simulink model "HANcoder_E407_GTSync_v3"  (R2018b)
settings: Solver=FixedStepDiscrete  StartTime=0.0  StopTime=1  FixedStep=0.01  RelTol=1e-3
PreLoadFcn:
  | librarySetup
  | eval([bdroot,'_startup']) %Calling [modelName]_startup.m
values from neighbouring files (symbols this model uses):
  frequency_IRQ = 100    [HANcoder_E407_GTSync_startup.m]    (also in HANcoder_E407_GTSync_v3_clean_startup.m = 99; HANcoder_E407_GTSync_v3_startup.m = 99)
  HANtuneOverride = Simulink.Parameter    [HANcoder_E407_GTSync_startup.m]    (also in HANcoder_E407_GTSync_v3_clean_startup.m; HANcoder_E407_GTSync_v3_startup.m)
  LED_ticks_toggle = 10000    [HANcoder_E407_GTSync_startup.m]    (also in HANcoder_E407_GTSync_v3_clean_startup.m; HANcoder_E407_GTSync_v3_startup.m)
  Master_Role = 1    [HANcoder_E407_GTSync_v3_clean_startup.m]    (also in HANcoder_E407_GTSync_v3_startup.m)
  matrix_rows = 2    [HANcoder_E407_GTSync_v3_clean_startup.m]    (also in HANcoder_E407_GTSync_v3_startup.m)
  Sync_ID = 1    [HANcoder_E407_GTSync_v3_clean_startup.m]    (also in HANcoder_E407_GTSync_v3_startup.m)
  time_difference_threshold = 500    [HANcoder_E407_GTSync_v3_clean_startup.m]    (also in HANcoder_E407_GTSync_v3_startup.m = 100)
  TM0 = 100    [HANcoder_E407_GTSync_v3_clean_startup.m]    (also in HANcoder_E407_GTSync_v3_startup.m = 0)
  TM1 = 20000    [HANcoder_E407_GTSync_v3_clean_startup.m]    (also in HANcoder_E407_GTSync_v3_startup.m = 25000)
  TM2 = 30000    [HANcoder_E407_GTSync_v3_clean_startup.m]    (also in HANcoder_E407_GTSync_v3_startup.m = 37500)
  TM3 = 40000    [HANcoder_E407_GTSync_v3_clean_startup.m]    (also in HANcoder_E407_GTSync_v3_startup.m)
  Vote1_ID = 12    [HANcoder_E407_GTSync_v3_clean_startup.m]    (also in HANcoder_E407_GTSync_v3_startup.m)
  Vote2_ID = 22    [HANcoder_E407_GTSync_v3_clean_startup.m]    (also in HANcoder_E407_GTSync_v3_startup.m)
  Vote3_ID = 32    [HANcoder_E407_GTSync_v3_clean_startup.m]    (also in HANcoder_E407_GTSync_v3_startup.m)
undefined symbols (not defined in the file or in its folder): votes
libraries: HANcoder_STM32_Target x20, simulink x3, simulink_extras x1
(part 2 of 2)

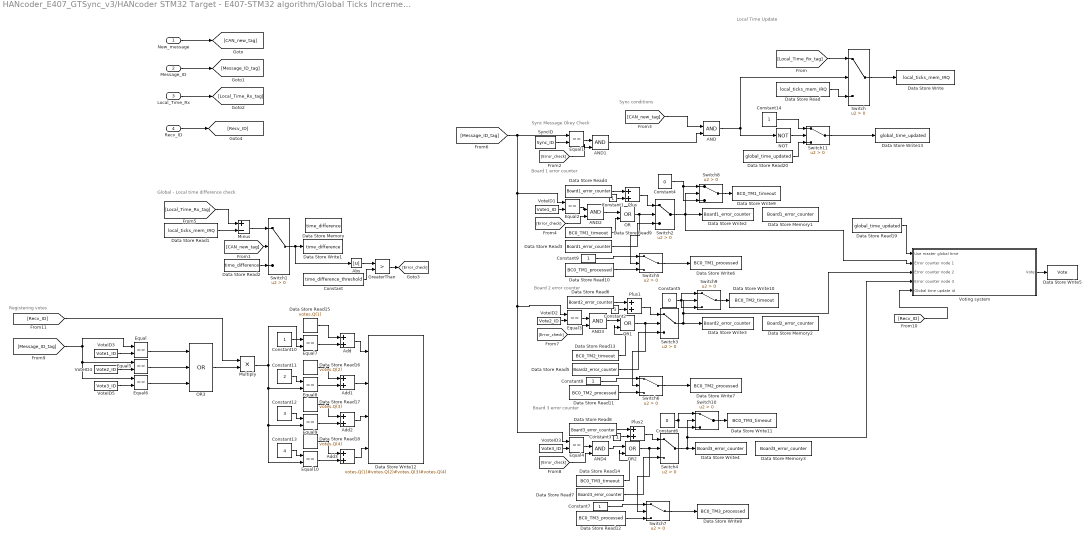
== system HANcoder_E407_GTSync_v3/HANcoder STM32 Target - E407-STM32 algorithm/Global Ticks Increment/CAN Management/Received message processing ==
  note: Registering votes
  note: Board 3 error counter
  note: Board 2 error counter
  note: Board 1 error counter
  note: Sync Message Okey Check
  note: Sync conditions
  note: Global - Local time difference check
  note: Local Time Update
  New_message : Inport
  Message_ID : Inport  Port=2
  Local_Time_Rx : Inport  Port=3
  Recv_ID : Inport  Port=4
  AND{,1..4} (5 alike) : Logic  IconShape=distinctive  AllPortsSameDT=off  OutDataTypeStr=boolean
  Abs : Abs
  Add{,1..3} (4 alike) : Sum
  Constant : Constant  Value=time_difference_threshold
  Constant{1..3,7..10,14} (8 alike) : Constant
  Constant11 : Constant  Value=2
  Constant12 : Constant  Value=3
  Constant13 : Constant  Value=4
  Constant4 : Constant  Value=0
  Constant5 : Constant  Value=0
  Constant6 : Constant  Value=0
  Data Store Memory : DataStoreMemory  DataStoreName=time_difference  ReadBeforeWriteMsg=warning  WriteAfterWriteMsg=warning  WriteAfterReadMsg=warning  ShowAdditionalParam=off
  Data Store Memory1 : DataStoreMemory  DataStoreName=Board1_error_counter  ReadBeforeWriteMsg=warning  WriteAfterWriteMsg=warning  WriteAfterReadMsg=warning  ShowAdditionalParam=off  OutMin=0  OutMax=4294967294  OutDataTypeStr=uint32
  Data Store Memory2 : DataStoreMemory  DataStoreName=Board2_error_counter  ReadBeforeWriteMsg=warning  WriteAfterWriteMsg=warning  WriteAfterReadMsg=warning  ShowAdditionalParam=off  OutMin=0  OutMax=4294967294  OutDataTypeStr=uint32
  Data Store Memory3 : DataStoreMemory  DataStoreName=Board3_error_counter  ReadBeforeWriteMsg=warning  WriteAfterWriteMsg=warning  WriteAfterReadMsg=warning  ShowAdditionalParam=off  OutMin=0  OutMax=4294967294  OutDataTypeStr=uint32
  Data Store Read : DataStoreRead  DataStoreName=local_ticks_mem_IRQ
  Data Store Read1 : DataStoreRead  DataStoreName=local_ticks_mem_IRQ
  Data Store Read10 : DataStoreRead  DataStoreName=BC0_TM1_processed
  Data Store Read11 : DataStoreRead  DataStoreName=BC0_TM2_processed
  Data Store Read12 : DataStoreRead  DataStoreName=BC0_TM3_processed
  Data Store Read13 : DataStoreRead  DataStoreName=BC0_TM2_timeout
  Data Store Read14 : DataStoreRead  DataStoreName=BC0_TM3_timeout
  Data Store Read15 : DataStoreRead  DataStoreName=votes  DataStoreElements=votes.Q(1)
  Data Store Read16 : DataStoreRead  DataStoreName=votes  DataStoreElements=votes.Q(2)
  Data Store Read17 : DataStoreRead  DataStoreName=votes  DataStoreElements=votes.Q(3)
  Data Store Read18 : DataStoreRead  DataStoreName=votes  DataStoreElements=votes.Q(4)
  Data Store Read19 : DataStoreRead  DataStoreName=global_time_updated
  Data Store Read2 : DataStoreRead  DataStoreName=time_difference
  Data Store Read20 : DataStoreRead  DataStoreName=global_time_updated
  Data Store Read3 : DataStoreRead  DataStoreName=Board1_error_counter
  Data Store Read4 : DataStoreRead  DataStoreName=Board1_error_counter
  Data Store Read5 : DataStoreRead  DataStoreName=Board2_error_counter
  Data Store Read6 : DataStoreRead  DataStoreName=Board2_error_counter
  Data Store Read7 : DataStoreRead  DataStoreName=Board3_error_counter
  Data Store Read8 : DataStoreRead  DataStoreName=Board3_error_counter
  Data Store Read9 : DataStoreRead  DataStoreName=BC0_TM1_timeout
  Data Store Write : DataStoreWrite  DataStoreName=local_ticks_mem_IRQ
  Data Store Write1 : DataStoreWrite  DataStoreName=time_difference
  Data Store Write10 : DataStoreWrite  DataStoreName=BC0_TM2_timeout
  Data Store Write11 : DataStoreWrite  DataStoreName=BC0_TM3_timeout
  Data Store Write12 : DataStoreWrite  DataStoreName=votes  DataStoreElements=votes.Q(1)#votes.Q(2)#votes.Q(3)#votes.Q(4)
  Data Store Write13 : DataStoreWrite  DataStoreName=global_time_updated
  Data Store Write2 : DataStoreWrite  DataStoreName=Board1_error_counter
  Data Store Write3 : DataStoreWrite  DataStoreName=Board2_error_counter
  Data Store Write4 : DataStoreWrite  DataStoreName=Board3_error_counter
  Data Store Write5 : DataStoreWrite  DataStoreName=Vote
  Data Store Write6 : DataStoreWrite  DataStoreName=BC0_TM1_processed
  Data Store Write7 : DataStoreWrite  DataStoreName=BC0_TM2_processed
  Data Store Write8 : DataStoreWrite  DataStoreName=BC0_TM3_processed
  Data Store Write9 : DataStoreWrite  DataStoreName=BC0_TM1_timeout
  Equal{,1..10} (11 alike) : RelationalOperator  Operator===  OutDataTypeStr=boolean  RndMeth=Simplest
  GreaterThan : RelationalOperator  Operator=>  OutDataTypeStr=boolean  RndMeth=Simplest
  Minus : Sum  Inputs=+-
  Multiply : Product
  NOT : Logic  Operator=NOT  IconShape=distinctive  AllPortsSameDT=off  OutDataTypeStr=boolean
  OR : Logic  Operator=OR  IconShape=distinctive  AllPortsSameDT=off  OutDataTypeStr=boolean
  OR1 : Logic  Operator=OR  IconShape=distinctive  AllPortsSameDT=off  OutDataTypeStr=boolean
  OR2 : Logic  Operator=OR  IconShape=distinctive  AllPortsSameDT=off  OutDataTypeStr=boolean
  OR3 : Logic  Operator=OR  Inputs=3  IconShape=distinctive  AllPortsSameDT=off  OutDataTypeStr=boolean
  Plus : Sum
  Plus1 : Sum
  Plus2 : Sum
  Switch{,1..11} (12 alike) : Switch  Criteria=u2 > Threshold
  SyncID : Constant  Value=Sync_ID
  VosteID3 : Constant  Value=Vote3_ID
  VoteID1 : Constant  Value=Vote1_ID
  VoteID2 : Constant  Value=Vote2_ID
  VoteID3 : Constant  Value=Vote1_ID
  VoteID4 : Constant  Value=Vote2_ID
  VoteID5 : Constant  Value=Vote3_ID
  Voting system : Subsystem
  wires:
  Data Store Read/1 -> Switch/3
  AND/1 -> Switch/2, NOT/1
  Switch/1 -> Data Store Write/1
  New_message/1 -> [CAN_new_tag]
  Message_ID/1 -> [Message_ID_tag]
  Local_Time_Rx/1 -> [Local_Time_Rx_tag]
  [Local_Time_Rx_tag] -> Switch/1
  AND1/1 -> AND/2
  [CAN_new_tag] -> AND/1
  [Local_Time_Rx_tag] -> Minus/1
  Data Store Read1/1 -> Minus/2
  Minus/1 -> Switch1/1
  [CAN_new_tag] -> Switch1/2
  Data Store Read2/1 -> Switch1/3
  SyncID/1 -> Equal1/2
  VoteID1/1 -> Equal2/2
  VoteID2/1 -> Equal3/2
  VosteID3/1 -> Equal4/2
  [Message_ID_tag] -> Equal4/1, Equal3/1, Equal2/1, Equal1/1
  Equal1/1 -> AND1/1
  Switch1/1 -> Abs/1, Data Store Write1/1
  Abs/1 -> GreaterThan/1
  Constant/1 -> GreaterThan/2
  [Error_check] -> AND1/2
  GreaterThan/1 -> [Error_check]
  Equal2/1 -> AND2/1
  [Error_check] -> AND2/2
  [Error_check] -> AND3/2
  Equal3/1 -> AND3/1
  [Error_check] -> AND4/2
  Equal4/1 -> AND4/1
  Data Store Read3/1 -> Switch2/3
  Data Store Read4/1 -> Plus/1
  Constant1/1 -> Plus/2
  Plus/1 -> Switch2/1
  Plus1/1 -> Switch3/1
  Constant2/1 -> Plus1/2
  Data Store Read6/1 -> Plus1/1
  Data Store Read5/1 -> Switch3/3
  Data Store Read7/1 -> Switch4/3
  Data Store Read8/1 -> Plus2/1
  Constant3/1 -> Plus2/2
  Plus2/1 -> Switch4/1
  Switch2/1 -> Voting system/2(Error counter node 1), Switch8/2, Data Store Write2/1
  Voting system/1(Vote) -> Data Store Write5/1
  [Recv_ID] -> Voting system/5(Global time update id)
  Recv_ID/1 -> [Recv_ID]
  Switch5/1 -> Data Store Write6/1
  AND3/1 -> OR1/1
  Switch6/1 -> Data Store Write7/1
  Data Store Read12/1 -> Switch7/3
  Switch7/1 -> Data Store Write8/1
  OR/1 -> Switch5/2, Switch2/2
  AND2/1 -> OR/1
  Data Store Read9/1 -> OR/2
  Constant4/1 -> Switch8/3, Switch8/1
  Switch8/1 -> Data Store Write9/1
  OR1/1 -> Switch6/2, Switch3/2
  Data Store Read13/1 -> OR1/2
  Switch3/1 -> Switch9/2, Voting system/3(Error counter node 2), Data Store Write3/1
  Switch9/1 -> Data Store Write10/1
  Constant5/1 -> Switch9/1, Switch9/3
  Switch10/1 -> Data Store Write11/1
  Switch4/1 -> Voting system/4(Error counter node 3), Switch10/2, Data Store Write4/1
  Constant6/1 -> Switch10/1, Switch10/3
  Data Store Read14/1 -> OR2/2
  OR2/1 -> Switch7/2, Switch4/2
  AND4/1 -> OR2/1
  Constant7/1 -> Switch7/1
  Data Store Read11/1 -> Switch6/3
  Constant8/1 -> Switch6/1
  Data Store Read10/1 -> Switch5/3
  Constant9/1 -> Switch5/1
  Equal/1 -> OR3/1
  VoteID3/1 -> Equal/2
  [Message_ID_tag] -> Equal/1, Equal6/1, Equal5/1
  VoteID4/1 -> Equal5/2
  Equal5/1 -> OR3/2
  VoteID5/1 -> Equal6/2
  Equal6/1 -> OR3/3
  [Recv_ID] -> Multiply/1
  OR3/1 -> Multiply/2
  Constant10/1 -> Equal7/1
  Equal7/1 -> Add/2
  Add/1 -> Data Store Write12/1
  Data Store Read15/1 -> Add/1
  Data Store Read16/1 -> Add1/1
  Constant11/1 -> Equal8/1
  Equal8/1 -> Add1/2
  Add1/1 -> Data Store Write12/2
  Equal9/1 -> Add2/2
  Data Store Read17/1 -> Add2/1
  Constant12/1 -> Equal9/1
  Add2/1 -> Data Store Write12/3
  Data Store Read18/1 -> Add3/1
  Multiply/1 -> Equal10/2, Equal9/2, Equal8/2, Equal7/2
  Equal10/1 -> Add3/2
  Constant13/1 -> Equal10/1
  Add3/1 -> Data Store Write12/4
  Data Store Read19/1 -> Voting system/1(Use master global time)
  NOT/1 -> Switch11/2
  Switch11/1 -> Data Store Write13/1
  Data Store Read20/1 -> Switch11/3
  Constant14/1 -> Switch11/1

== system HANcoder_E407_GTSync_v3/HANcoder STM32 Target - E407-STM32 algorithm/Global Ticks Increment/Send/CAN send ==
  In1 : Inport
  In2 : Inport  Port=2
  In3 : Inport  Port=3
  In4 : Inport  Port=4
  In5 : Inport  Port=5
  In6 : Inport  Port=6
  In7 : Inport  Port=7
  In8 : Inport  Port=8
  In9 : Inport  Port=9
  S-Function : M-S-Function  FunctionName=sfcn_can_send  Parameters=tsamp, canBus, frameType, inputNumber, dataType, byteOrder
  wires:
  In1/1 -> S-Function/1
  In2/1 -> S-Function/2
  In3/1 -> S-Function/3
  In4/1 -> S-Function/4
  In5/1 -> S-Function/5
  In6/1 -> S-Function/6
  In7/1 -> S-Function/7
  In8/1 -> S-Function/8
  In9/1 -> S-Function/9

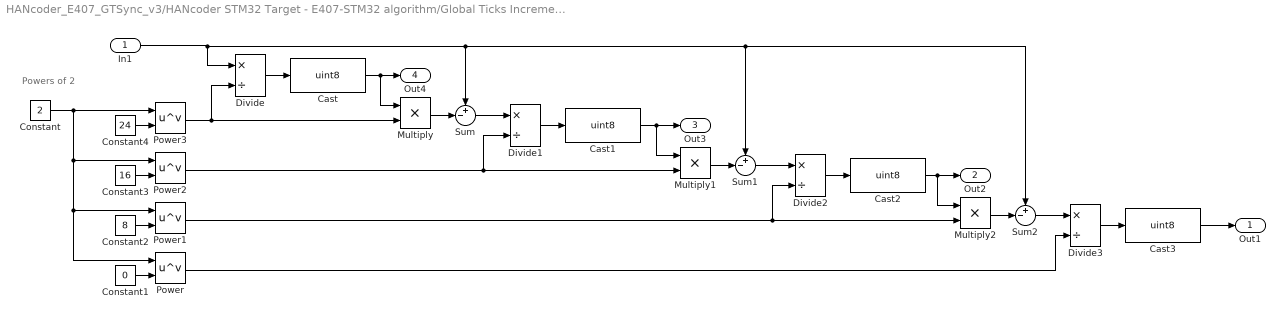
== system HANcoder_E407_GTSync_v3/HANcoder STM32 Target - E407-STM32 algorithm/Global Ticks Increment/Send/UINT32 to UINT8 ==
  note: Powers of 2
  In1 : Inport
  Cast{,1..3} (4 alike) : DataTypeConversion  OutDataTypeStr=uint8
  Constant : Constant  Value=2
  Constant1 : Constant  Value=0
  Constant2 : Constant  Value=8
  Constant3 : Constant  Value=16
  Constant4 : Constant  Value=24
  Divide{,1..3} (4 alike) : Product  Inputs=*/
  Multiply : Product
  Multiply1 : Product
  Multiply2 : Product
  Power{,1..3} (4 alike) : Math  Operator=pow  SaturateOnIntegerOverflow=on
  Sum : Sum  Inputs=+-|
  Sum1 : Sum  Inputs=+-|
  Sum2 : Sum  Inputs=+-|
  Out1 : Outport
  Out2 : Outport  Port=2
  Out3 : Outport  Port=3
  Out4 : Outport  Port=4
  wires:
  Constant2/1 -> Power1/2
  Constant3/1 -> Power2/2
  Constant4/1 -> Power3/2
  Power2/1 -> Multiply1/2, Divide1/2
  Constant1/1 -> Power/2
  Power3/1 -> Divide/2, Multiply/2
  Constant/1 -> Power/1, Power1/1, Power2/1, Power3/1
  Divide/1 -> Cast/1
  Cast/1 -> Multiply/1, Out4/1
  Multiply/1 -> Sum/2
  Divide1/1 -> Cast1/1
  Sum/1 -> Divide1/1
  Cast1/1 -> Out3/1, Multiply1/1
  Multiply1/1 -> Sum1/2
  Multiply2/1 -> Sum2/2
  Cast2/1 -> Out2/1, Multiply2/1
  Divide2/1 -> Cast2/1
  Power1/1 -> Multiply2/2, Divide2/2
  Sum1/1 -> Divide2/1
  Sum2/1 -> Divide3/1
  In1/1 -> Sum1/1, Sum2/1, Sum/1, Divide/1
  Power/1 -> Divide3/2
  Divide3/1 -> Cast3/1
  Cast3/1 -> Out1/1

== system HANcoder_E407_GTSync_v3/HANcoder STM32 Target - E407-STM32 algorithm/Global Ticks Increment/CAN Management/CAN Recieve/CAN receive ==
  In1 : Inport
  Enabled Subsystem : Subsystem  TreatAsAtomicUnit=on
  S-Function : M-S-Function  FunctionName=sfcn_can_receive  Parameters=tsamp, canBus, outputNumber, dataType, byteOrder
  Out1 : Outport
  Out2 : Outport  Port=2
  Out3 : Outport  Port=3
  Out4 : Outport  Port=4
  Out5 : Outport  Port=5
  Out6 : Outport  Port=6
  Out7 : Outport  Port=7
  Out8 : Outport  Port=8
  Out9 : Outport  Port=9
  wires:
  S-Function/9 -> Enabled Subsystem/8(In8)
  S-Function/4 -> Enabled Subsystem/3(In3)
  S-Function/5 -> Enabled Subsystem/4(In4)
  S-Function/8 -> Enabled Subsystem/7(In7)
  S-Function/7 -> Enabled Subsystem/6(In6)
  S-Function/6 -> Enabled Subsystem/5(In5)
  Enabled Subsystem/8(Out8) -> Out9/1
  Enabled Subsystem/7(Out7) -> Out8/1
  Enabled Subsystem/6(Out6) -> Out7/1
  Enabled Subsystem/5(Out5) -> Out6/1
  Enabled Subsystem/4(Out4) -> Out5/1
  Enabled Subsystem/3(Out3) -> Out4/1
  Enabled Subsystem/2(Out2) -> Out3/1
  Enabled Subsystem/1(Out1) -> Out2/1
  S-Function/3 -> Enabled Subsystem/2(In2)
  S-Function/2 -> Enabled Subsystem/1(In1)
  S-Function/1 -> Out1/1, Enabled Subsystem/Enable
  In1/1 -> S-Function/1

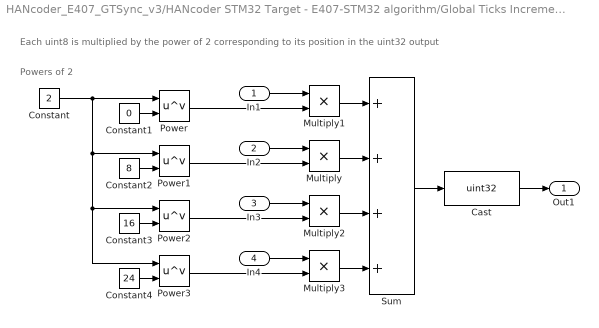
== system HANcoder_E407_GTSync_v3/HANcoder STM32 Target - E407-STM32 algorithm/Global Ticks Increment/CAN Management/CAN Recieve/UINT8 to UINT32 ==
  note: Each uint8 is multiplied by the power of 2 corresponding to its position in the uint32 output
  note: Powers of 2
  In1 : Inport
  In2 : Inport  Port=2
  In3 : Inport  Port=3
  In4 : Inport  Port=4
  Cast : DataTypeConversion  OutDataTypeStr=uint32
  Constant : Constant  Value=2
  Constant1 : Constant  Value=0
  Constant2 : Constant  Value=8
  Constant3 : Constant  Value=16
  Constant4 : Constant  Value=24
  Multiply{,1..3} (4 alike) : Product
  Power{,1..3} (4 alike) : Math  Operator=pow  SaturateOnIntegerOverflow=on
  Sum : Sum  Inputs=++++
  Out1 : Outport
  wires:
  Cast/1 -> Out1/1
  Sum/1 -> Cast/1
  In1/1 -> Multiply1/1
  In2/1 -> Multiply/1
  In3/1 -> Multiply2/1
  In4/1 -> Multiply3/1
  Constant/1 -> Power3/1, Power2/1, Power1/1, Power/1
  Constant1/1 -> Power/2
  Constant2/1 -> Power1/2
  Constant3/1 -> Power2/2
  Constant4/1 -> Power3/2
  Power/1 -> Multiply1/2
  Power1/1 -> Multiply/2
  Power2/1 -> Multiply2/2
  Power3/1 -> Multiply3/2
  Multiply3/1 -> Sum/4
  Multiply2/1 -> Sum/3
  Multiply/1 -> Sum/2
  Multiply1/1 -> Sum/1

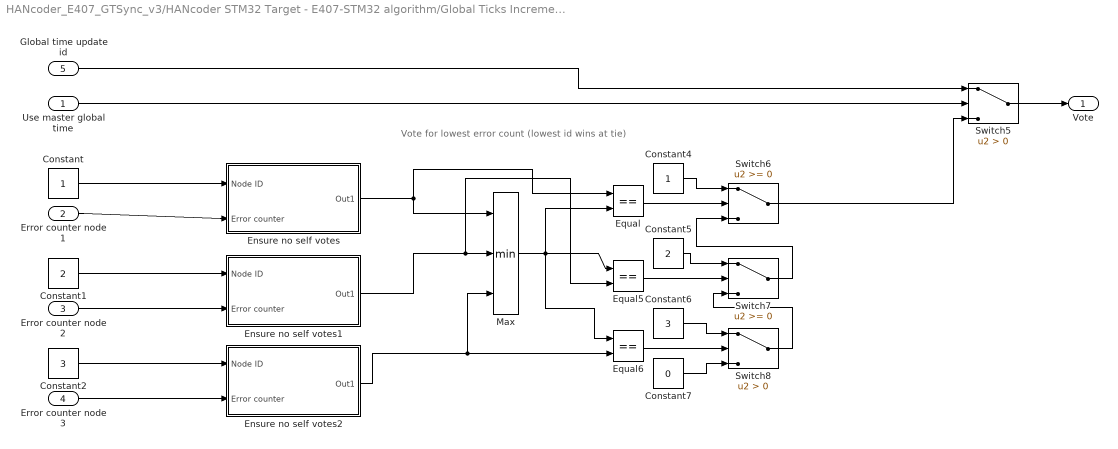
== system HANcoder_E407_GTSync_v3/HANcoder STM32 Target - E407-STM32 algorithm/Global Ticks Increment/CAN Management/Received message processing/Voting system ==
  note: Vote for lowest error count (lowest id wins at tie)
  Use master global time : Inport
  Error counter node 1 : Inport  Port=2
  Error counter node 2 : Inport  Port=3
  Error counter node 3 : Inport  Port=4
  Global time update id : Inport  Port=5
  Constant : Constant
  Constant1 : Constant  Value=2
  Constant2 : Constant  Value=3
  Constant4 : Constant
  Constant5 : Constant  Value=2
  Constant6 : Constant  Value=3
  Constant7 : Constant  Value=0
  Ensure no self votes : Subsystem
  Ensure no self votes1 : Subsystem
  Ensure no self votes2 : Subsystem
  Equal : RelationalOperator  Operator===  OutDataTypeStr=boolean  RndMeth=Simplest
  Equal5 : RelationalOperator  Operator===  OutDataTypeStr=boolean  RndMeth=Simplest
  Equal6 : RelationalOperator  Operator===  OutDataTypeStr=boolean  RndMeth=Simplest
  Max : MinMax  Inputs=3
  Switch5 : Switch  Criteria=u2 > Threshold
  Switch6 : Switch
  Switch7 : Switch
  Switch8 : Switch  Criteria=u2 > Threshold
  Vote : Outport
  wires:
  Equal5/1 -> Switch7/2
  Ensure no self votes1/1(Out1) -> Equal5/2, Max/2
  Constant5/1 -> Switch7/1
  Equal6/1 -> Switch8/2
  Ensure no self votes2/1(Out1) -> Max/3, Equal6/2
  Switch7/1 -> Switch6/3
  Switch5/1 -> Vote/1
  Max/1 -> Equal/2, Equal5/1, Equal6/1
  Switch6/1 -> Switch5/3
  Switch8/1 -> Switch7/3
  Constant7/1 -> Switch8/3
  Equal/1 -> Switch6/2
  Constant6/1 -> Switch8/1
  Constant4/1 -> Switch6/1
  Global time update id/1 -> Switch5/1
  Use master global time/1 -> Switch5/2
  Ensure no self votes/1(Out1) -> Equal/1, Max/1
  Constant/1 -> Ensure no self votes/1(Node ID)
  Error counter node 1/1 -> Ensure no self votes/2(Error counter)
  Error counter node 2/1 -> Ensure no self votes1/2(Error counter)
  Constant1/1 -> Ensure no self votes1/1(Node ID)
  Error counter node 3/1 -> Ensure no self votes2/2(Error counter)
  Constant2/1 -> Ensure no self votes2/1(Node ID)

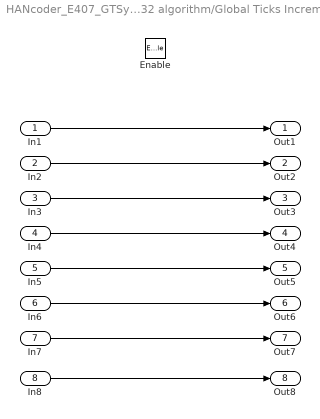
== system HANcoder_E407_GTSync_v3/HANcoder STM32 Target - E407-STM32 algorithm/Global Ticks Increment/CAN Management/CAN Recieve/CAN receive/Enabled Subsystem ==
  In1 : Inport
  In2 : Inport  Port=2
  In3 : Inport  Port=3
  In4 : Inport  Port=4
  In5 : Inport  Port=5
  In6 : Inport  Port=6
  In7 : Inport  Port=7
  In8 : Inport  Port=8
  Enable : EnablePort
  Out1 : Outport
  Out2 : Outport  Port=2
  Out3 : Outport  Port=3
  Out4 : Outport  Port=4
  Out5 : Outport  Port=5
  Out6 : Outport  Port=6
  Out7 : Outport  Port=7
  Out8 : Outport  Port=8
  wires:
  In8/1 -> Out8/1
  In7/1 -> Out7/1
  In6/1 -> Out6/1
  In5/1 -> Out5/1
  In4/1 -> Out4/1
  In3/1 -> Out3/1
  In2/1 -> Out2/1
  In1/1 -> Out1/1

== system HANcoder_E407_GTSync_v3/HANcoder STM32 Target - E407-STM32 algorithm/Global Ticks Increment/CAN Management/Received message processing/Voting system/Ensure no self votes ==
  Node ID : Inport
  Error counter : Inport  Port=2
  Data Store Read : DataStoreRead  DataStoreName=Board_ID
  Equal1 : RelationalOperator  Operator===  OutDataTypeStr=boolean  RndMeth=Simplest
  MAX error count : Constant  Value=4294967295  OutDataTypeStr=uint32
  Switch : Switch  Criteria=u2 > Threshold
  Out1 : Outport
  wires:
  Equal1/1 -> Switch/2
  Data Store Read/1 -> Equal1/2
  MAX error count/1 -> Switch/1
  Switch/1 -> Out1/1
  Error counter/1 -> Switch/3
  Node ID/1 -> Equal1/1

== system HANcoder_E407_GTSync_v3/HANcoder STM32 Target - E407-STM32 algorithm/Global Ticks Increment/CAN Management/Received message processing/Voting system/Ensure no self votes1 ==
  Node ID : Inport
  Error counter : Inport  Port=2
  Data Store Read : DataStoreRead  DataStoreName=Board_ID
  Equal1 : RelationalOperator  Operator===  OutDataTypeStr=boolean  RndMeth=Simplest
  MAX error count : Constant  Value=4294967295  OutDataTypeStr=uint32
  Switch : Switch  Criteria=u2 > Threshold
  Out1 : Outport
  wires:
  Equal1/1 -> Switch/2
  Data Store Read/1 -> Equal1/2
  MAX error count/1 -> Switch/1
  Switch/1 -> Out1/1
  Error counter/1 -> Switch/3
  Node ID/1 -> Equal1/1

== system HANcoder_E407_GTSync_v3/HANcoder STM32 Target - E407-STM32 algorithm/Global Ticks Increment/CAN Management/Received message processing/Voting system/Ensure no self votes2 ==
  Node ID : Inport
  Error counter : Inport  Port=2
  Data Store Read : DataStoreRead  DataStoreName=Board_ID
  Equal1 : RelationalOperator  Operator===  OutDataTypeStr=boolean  RndMeth=Simplest
  MAX error count : Constant  Value=4294967295  OutDataTypeStr=uint32
  Switch : Switch  Criteria=u2 > Threshold
  Out1 : Outport
  wires:
  Equal1/1 -> Switch/2
  Data Store Read/1 -> Equal1/2
  MAX error count/1 -> Switch/1
  Switch/1 -> Out1/1
  Error counter/1 -> Switch/3
  Node ID/1 -> Equal1/1

== stateflow chart HANcoder_E407_GTSync_v3/HANcoder STM32 Target - E407-STM32 algorithm/Global Ticks Increment/Function-Call Subsystem/Even_Tick ==
  settings: initializeOutput=1
  state Even_tick
    if (mod(current_tick,2)==0)
    active_flag = 1;
    end
  state Rise_edge
    send(rise_edge_at_even)
  (default) -> Even_tick
  Even_tick -> Rise_edge : [active_flag == 1]
  data: current_tick input; active_flag local =0
  events: rise_edge_at_even output EITHER_EDGE_EVENT

== stateflow chart HANcoder_E407_GTSync_v3/HANcoder STM32 Target - E407-STM32 algorithm/Global Ticks Increment/Function-Call Subsystem/Odd_Tick ==
  settings: initializeOutput=1
  state Odd_tick
    if (mod(current_tick,2)==1)
    active_flag = 1;
    end
  state Rise_edge
    send(rise_edge_at_odd)
  (default) -> Odd_tick
  Odd_tick -> Rise_edge : [active_flag == 1]
  data: current_tick input; active_flag local =0
  events: rise_edge_at_odd output EITHER_EDGE_EVENT

== stateflow chart HANcoder_E407_GTSync_v3/HANcoder STM32 Target - E407-STM32 algorithm/Global Ticks Increment/Function-Call Subsystem/Check_Reset_Idle_Time ==
  settings: initializeOutput=1
  state Check_WKUP
    if WKUP_state
    send(WKUP_CAN)
    end
  (default) -> Check_WKUP
  data: WKUP_state input
  events: WKUP_CAN output FUNCTION_CALL_EVENT

== stateflow chart HANcoder_E407_GTSync_v3/HANcoder STM32 Target - E407-STM32 algorithm/Global Ticks Increment/CAN Management/Check_Reset_Idle_Time ==
  settings: initializeOutput=1
  state Check_Condition
    if condition
    send(send_function_call)
    end
  (default) -> Check_Condition
  data: condition input
  events: send_function_call output FUNCTION_CALL_EVENT
